simulink model "Receive_Realsense"  (R2023a)
settings: Solver=VariableStepAuto  StartTime=0.0  StopTime=inf  FixedStep=0.01  RelTol=1e-3
undefined symbols (not defined in the file or in its folder): gray
settings Model: Creator=LG gram 17 - HW dev  LastModifiedBy=LG gram 17 - HW dev

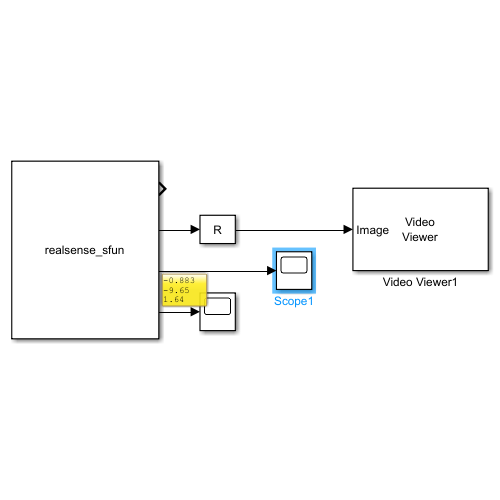
[thumbnail: Simulink's stored preview of the top-level diagram]
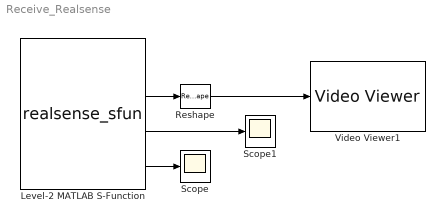
== system Receive_Realsense ==
  Level-2 MATLAB S-Function : M-S-Function  FunctionName=realsense_sfun
  Reshape : Reshape  OutputDimensionality=Customize  OutputDimensions=[720 1280 3]
  Scope : Scope
  Scope1 : Scope
  Video Viewer1 : VideoViewer  colormapValue=gray(256)  FigPos=[564.333333333333 500.666666666667 675.333333333333 398]
  wires:
  Reshape/1 -> Video Viewer1/1
  Level-2 MATLAB S-Function/4 -> Scope/1
  Level-2 MATLAB S-Function/3 -> Scope1/1
  Level-2 MATLAB S-Function/2 -> Reshape/1
